simulink model "trajectory_servo_control"  (R2024a)
settings: Solver=FixedStepAuto  StartTime=0.0  StopTime=inf  FixedStep=0.005  RelTol=1e-3  EnableMultiTasking=on
libraries: arduinolib x7, simulink x5
settings Model: ExtModeTrigDuration=2  Creator=ibrahim elshami  LastModifiedBy=Phoebe Emil
settings SolverCC: AutoInsertRateTranBlk=on
settings OptimizationCC: EnhancedBackFolding=on  PassReuseOutputArgsAs=Individual arguments  ZeroExternalMemoryAtStartup=off  ZeroInternalMemoryAtStartup=off  MaxStackSize=64  OptimizeBlockOrder=speed  DifferentSizesBufferReuse=on  OptimizationCustomize=off  EfficientTunableParamExpr=on
settings DebuggingCC: ParameterTunabilityLossMsg=error
settings HardwareCC: ProdBitPerPointer=32  ProdBitPerSizeT=32  ProdBitPerPtrDiffT=32  ProdLargestAtomicInteger=Long  ProdLargestAtomicFloat=Double  ProdWordSize=32  ProdHWDeviceType=ARM Compatible->ARM Cortex
settings SFSimCC: MATLABDynamicMemAlloc=off
settings RTWCC: Description=Embedded Coder  SystemTargetFile=ert.tlc  HardwareBoard=ESP32-WROOM(Arduino Compatible)  TLCOptions="-aInlineSetEventsForThisBaseRateFcn=TLC_FALSE -aSuppressMultiTaskScheduler=TLC_FALSE  -aRateBasedStepFcn=0"  TemplateMakefile=ert_default_tmf  Toolchain=ESP32  BuildConfiguration=Faster Runs
settings CodeAppCC: ForceParamTrailComments=on  IgnoreCustomStorageClasses=off  OperatorAnnotations=on  SimulinkDataObjDesc=on  SFDataObjDesc=on  InsertBlockDesc=on
settings ERTTargetCC: SupportContinuousTime=on  SupportVariableSizeSignals=on  ExtModeTransport=3  ExtModeStaticAlloc=on  ExtModeAutomaticAllocSize=off  ExtModeStaticAllocSize=65536  ExtModeMexFile=ext_xcp  ExtModeIntrfLevel=Level2 - Open

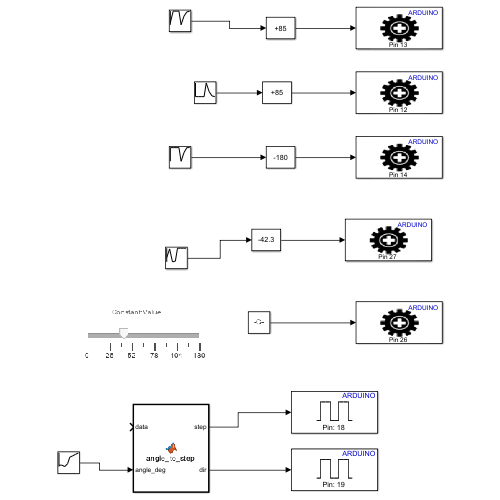
[thumbnail: Simulink's stored preview of the top-level diagram]
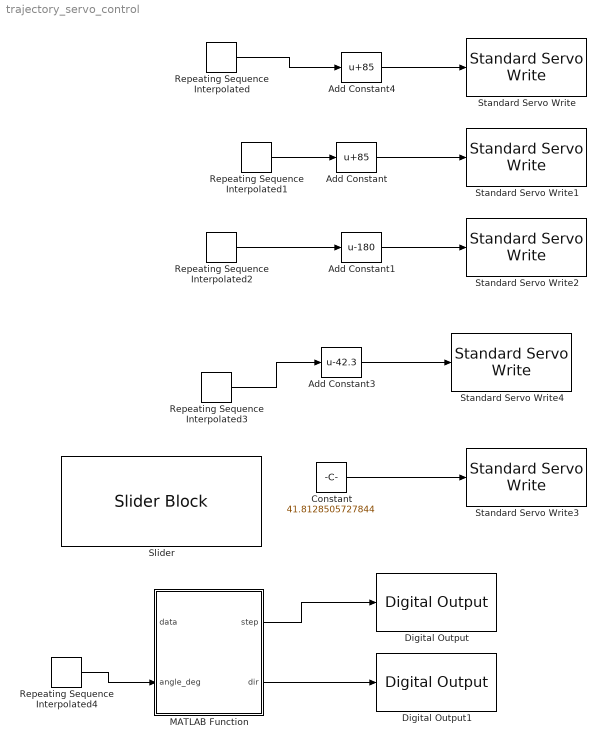
== system trajectory_servo_control ==
  Add Constant : Bias  Bias=85  SaturateOnIntegerOverflow=off
  Add Constant1 : Bias  Bias=-180  SaturateOnIntegerOverflow=off
  Add Constant3 : Bias  Bias=-42.3  SaturateOnIntegerOverflow=off
  Add Constant4 : Bias  Bias=85  SaturateOnIntegerOverflow=off
  Constant : Constant  Value=41.8128505727844
  Digital Output : arduinolib/Digital Output  pinNumber=18  Direction=output  blockPlatform=arduino
  Digital Output1 : arduinolib/Digital Output  pinNumber=19  Direction=output  blockPlatform=arduino
  MATLAB Function : MATLAB Function  TreatAsAtomicUnit=on
  Repeating Sequence Interpolated : simulink/Sources/Repeating Sequence Interpolated  OutValues=pj2  TimeValues=[0 1 2 3 4 5 6 7].'  LookUpMeth=Interpolation-Use End Values  tsamp=0.01  OutMin=[]  OutMax=[]  OutDataTypeStr=double  OutputDataTypeScalingMode=double  OutDataType=fixdt(0,8)  OutScaling=2^-10
  Repeating Sequence Interpolated1 : simulink/Sources/Repeating Sequence Interpolated  OutValues=pj3  TimeValues=[0 1 2 3 4 5 6 7].'  LookUpMeth=Interpolation-Use End Values  tsamp=0.01  OutMin=[]  OutMax=[]  OutDataTypeStr=double  OutputDataTypeScalingMode=double  OutDataType=fixdt(0,8)  OutScaling=2^-10
  Repeating Sequence Interpolated2 : simulink/Sources/Repeating Sequence Interpolated  OutValues=pj4  TimeValues=[0 1 2 3 4 5 6 7].'  LookUpMeth=Interpolation-Use End Values  tsamp=0.01  OutMin=[]  OutMax=[]  OutDataTypeStr=double  OutputDataTypeScalingMode=double  OutDataType=fixdt(0,8)  OutScaling=2^-10
  Repeating Sequence Interpolated3 : simulink/Sources/Repeating Sequence Interpolated  OutValues=pj5  TimeValues=[0 1 2 3 4 5 6 7].'  LookUpMeth=Interpolation-Use End Values  tsamp=0.01  OutMin=[]  OutMax=[]  OutDataTypeStr=double  OutputDataTypeScalingMode=double  OutDataType=fixdt(0,8)  OutScaling=2^-10
  Repeating Sequence Interpolated4 : simulink/Sources/Repeating Sequence Interpolated  OutValues=pj1  TimeValues=[0 1 2 3 4 5 6 7].'  LookUpMeth=Interpolation-Use End Values  tsamp=0.01  OutMin=[]  OutMax=[]  OutDataTypeStr=double  OutputDataTypeScalingMode=double  OutDataType=fixdt(0,8)  OutScaling=2^-10
  Slider : SliderBlock  ScaleMax=130
  Standard Servo Write : arduinolib/Standard Servo Write  pinNumber=13  ServoIndex=0  blockPlatform=ARDUINO
  Standard Servo Write1 : arduinolib/Standard Servo Write  pinNumber=12  ServoIndex=1  blockPlatform=ARDUINO
  Standard Servo Write2 : arduinolib/Standard Servo Write  pinNumber=14  ServoIndex=2  blockPlatform=ARDUINO
  Standard Servo Write3 : arduinolib/Standard Servo Write  pinNumber=26  ServoIndex=3  blockPlatform=ARDUINO
  Standard Servo Write4 : arduinolib/Standard Servo Write  pinNumber=27  ServoIndex=4  blockPlatform=ARDUINO
  wires:
  Add Constant4/1 -> Standard Servo Write/1
  Add Constant/1 -> Standard Servo Write1/1
  Add Constant1/1 -> Standard Servo Write2/1
  Add Constant3/1 -> Standard Servo Write4/1
  MATLAB Function/1(step) -> Digital Output/1
  MATLAB Function/2(dir) -> Digital Output1/1
  Repeating Sequence Interpolated4/1 -> MATLAB Function/2(angle_deg)
  Repeating Sequence Interpolated3/1 -> Add Constant3/1
  Repeating Sequence Interpolated2/1 -> Add Constant1/1
  Repeating Sequence Interpolated1/1 -> Add Constant/1
  Repeating Sequence Interpolated/1 -> Add Constant4/1
  Constant/1 -> Standard Servo Write3/1

== matlab function trajectory_servo_control/MATLAB Function ==
  data: data input; angle_deg input; step output; dir output
function [step, dir] = angle_to_step(data, angle_deg)
%#codegen

% ── Motor parameters ──────────────────────────────────
STEPS_PER_REV = 200;    % steps per full revolution
% Solver fixed step size must equal HALF_PERIOD
% e.g. 5000 us = 0.005 s  →  set solver step = 0.005

% ── Persistent state ──────────────────────────────────
persistent count target last_angle pulse_phase
if isempty(count)
    count       = int32(0);
    target      = int32(0);
    last_angle  = 0;
    pulse_phase = false;   % false = HIGH phase, true = LOW phase
end

% ── Direction ─────────────────────────────────────────
dir = angle_deg >= 0;

% ── Load new target when angle input changes ──────────
if angle_deg ~= last_angle
    target      = int32(round(abs(angle_deg) * STEPS_PER_REV / 360));
    count       = int32(0);
    last_angle  = angle_deg;
    pulse_phase = false;
end

% ── Two-phase pulse generation ────────────────────────
if count < target
    if ~pulse_phase
        % Phase 1: drive STEP HIGH for one solver tick (5000 us)
        step        = true;
        pulse_phase = true;    % next tick → go LOW
    else
        % Phase 2: drive STEP LOW for one solver tick (5000 us)
        step        = false;
        pulse_phase = false;   % next tick → next step
        count       = count + int32(1);   % count AFTER full pulse
    end
else
    step        = false;
    pulse_phase = false;
end
